simulink model "tp1ej1pG"  (R2024a)
settings: Solver=VariableStepAuto  StartTime=0.0  StopTime=20.0  RelTol=1e-3
settings Model: Creator=fab  LastModifiedBy=fab

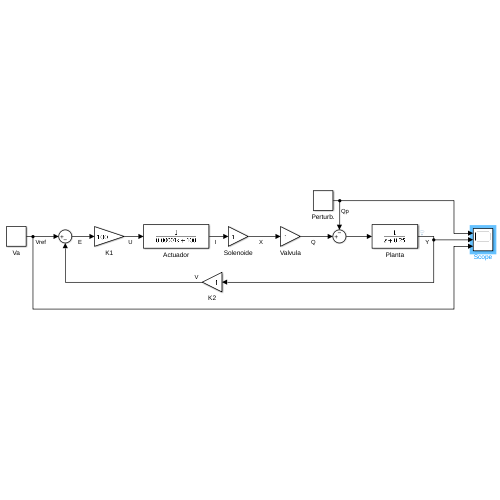
[thumbnail: Simulink's stored preview of the top-level diagram]
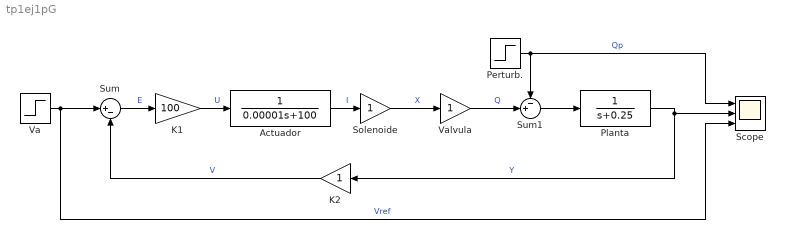
== system tp1ej1pG ==
  Actuador : TransferFcn  Denominator=[0.00001 100]
  K1 : Gain  Gain=100
  K2 : Gain
  Perturb. : Step  Time=10  After=2  SampleTime=0
  Planta : TransferFcn  Denominator=[1 0.25]
  Scope : Scope  NumInputPorts=3
  Solenoide : Gain
  Sum : Sum  Inputs=|+-
  Sum1 : Sum  Inputs=-+|
  Va : Step  After=10  SampleTime=0
  Valvula : Gain
  wires:
  Va/1 -> Scope/3, Sum/1  "Vref"
  Sum/1 -> K1/1  "E"
  K1/1 -> Actuador/1  "U"
  Actuador/1 -> Solenoide/1  "I"
  Solenoide/1 -> Valvula/1  "X"
  Valvula/1 -> Sum1/2  "Q"
  K2/1 -> Sum/2  "V"
  Planta/1 -> K2/1, Scope/2  "Y"
  Sum1/1 -> Planta/1
  Perturb./1 -> Scope/1, Sum1/1  "Qp"
